simulink model "lab3"  (R2021b)
settings: Solver=VariableStepAuto  StartTime=0.0  StopTime=700  RelTol=1e-3
undefined symbols (not defined in the file): c, J, kb, kt, L, R
libraries: simulink x5, slpidlib x1
settings Model: Creator=Venik  LastModifiedBy=Venik

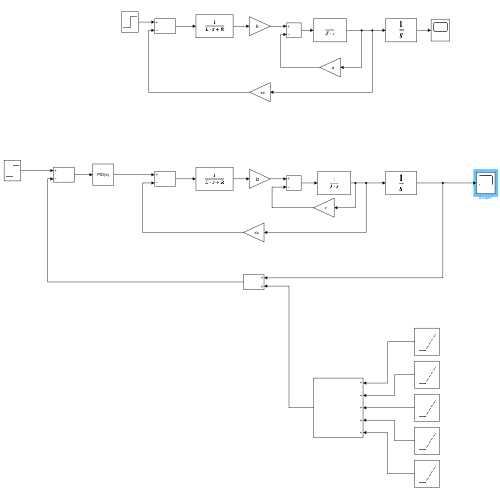
[thumbnail: Simulink's stored preview of the top-level diagram]
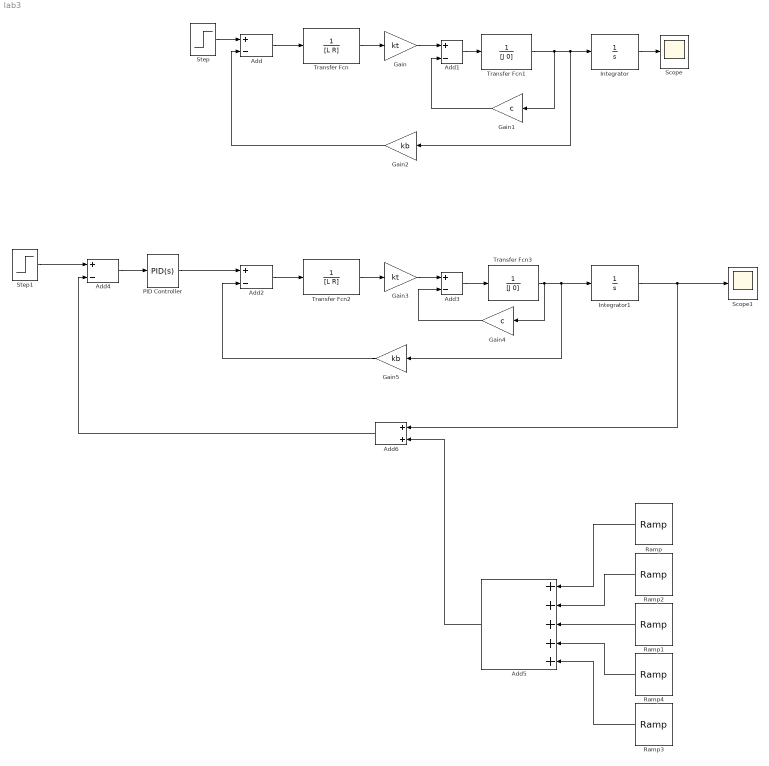
== system lab3 ==
  Add{,1..4} (5 alike) : Sum  Inputs=+-
  Add5 : Sum  Inputs=+++++
  Add6 : Sum
  Gain : Gain  Gain=kt
  Gain1 : Gain  Gain=c
  Gain2 : Gain  Gain=kb
  Gain3 : Gain  Gain=kt
  Gain4 : Gain  Gain=c
  Gain5 : Gain  Gain=kb
  Integrator : Integrator
  Integrator1 : Integrator
  PID Controller : slpidlib/PID Controller  Controller=PID  Form=Parallel  TimeDomain=Continuous-time  UseExternalTs=off  SampleTime=-1  IntegratorMethod=Forward Euler  FilterMethod=Forward Euler  ControllerParametersSource=internal  P=2  I=0.1  D=10  UseFilter=on  N=100  TunerSelectOption=Transfer Function Based (PID Tuner App)  InitialConditionSource=internal  InitialConditionForIntegrator=0  InitialConditionForFilter=0  DifferentiatorICPrevScaledInput=0  ExternalReset=none  TrackingMode=off  Kt=1  LimitOutput=off  SatLimitsSource=internal  UpperSaturationLimit=inf  LowerSaturationLimit=-inf  LinearizeAsGain=on  AntiWindupMode=none  Kb=1  POutMin=[]  POutMax=[]  IOutMin=[]  IOutMax=[]  DOutMin=[]  DOutMax=[]  NOutMin=[]  NOutMax=[]  SumOutMin=[]  SumOutMax=[]  SaturationOutMin=[]  SaturationOutMax=[]  PParamMin=[]  PParamMax=[]  IParamMin=[]  IParamMax=[]  DParamMin=[]  DParamMax=[]  NParamMin=[]  NParamMax=[]  KbParamMin=[]  KbParamMax=[]  KtParamMin=[]  KtParamMax=[]  KbOutMin=[]  KbOutMax=[]  KtOutMin=[]  KtOutMax=[]  IntegratorOutMin=[]  IntegratorOutMax=[]  FilterOutMin=[]  FilterOutMax=[]  SumI1OutMin=[]  SumI1OutMax=[]  SumI2OutMin=[]  SumI2OutMax=[]  SumI3OutMin=[]  SumI3OutMax=[]  SumI4OutMin=[]  SumI4OutMax=[]  SumDOutMin=[]  SumDOutMax=[]  DifferentiatorOutMin=[]  DifferentiatorOutMax=[]  FilterDiffOutCoefMin=[]  FilterDiffOutCoefMax=[]  ReciprocalOutMin=[]  ReciprocalOutMax=[]  SumDenOutMin=[]  SumDenOutMax=[]  SumNumOutMin=[]  SumNumOutMax=[]  DivideOutMin=[]  DivideOutMax=[]  UdiffTsProdOutMin=[]  UdiffTsProdOutMax=[]  NTsProdOutMin=[]  NTsProdOutMax=[]  UintegralTsProdOutMin=[]  UintegralTsProdOutMax=[]  UngainTsProdOutMin=[]  UngainTsProdOutMax=[]  IntegratorContinuousStateAttributes=''  IntegratorStateMustResolveToSignalObject=off  IntegratorRTWStateStorageClass=Auto  FilterContinuousStateAttributes=''  FilterStateMustResolveToSignalObject=off  FilterRTWStateStorageClass=Auto  ParallelPVariant=InternalParameters  IdealPVariant=Disabled  IVariant=InternalParameters  DVariant=InternalParameters  IntegratorVariant=Continuous  SatVariant=Disabled  AWVariant=Passthrough  PCopyVariant=Disabled  TRVariant=Disabled  FdbkBlocksVariant=Forward  IdealPFdbkVariant=Disabled  SatFdbkVariant=Disabled  DerivativeFilterVariant=ContFilter  NVariant=InternalParameters  NCopyVariant=Disabled  FilterICVariant=InternalICsFilter  IntegratorICVariant=InternalICs  ExternalResetVariant=Disabled  TRSumVariant=Passthrough  SumFdbkVariant=Disabled  SumVariant=Sum_PID  TsampFilterVariant=InternalTs  TsampNgainVariant=Passthrough  TsampIntegralVariant=Passthrough  ExternalSaturationOutDataTypeStr=Inherit: Same as second input
  Ramp : simulink/Sources/Ramp  slope=0  start=0  InitialOutput=0
  Ramp1 : simulink/Sources/Ramp  slope=-0.2  start=170  InitialOutput=0
  Ramp2 : simulink/Sources/Ramp  slope=0.2  start=150  InitialOutput=0
  Ramp3 : simulink/Sources/Ramp  slope=0.1  start=350  InitialOutput=0
  Ramp4 : simulink/Sources/Ramp  slope=-0.1  start=300  InitialOutput=0
  Scope : Scope
  Scope1 : Scope
  Step : Step  After=3  SampleTime=0
  Step1 : Step  After=3  SampleTime=0
  Transfer Fcn : TransferFcn  Denominator=[L R]
  Transfer Fcn1 : TransferFcn  Denominator=[J 0]
  Transfer Fcn2 : TransferFcn  Denominator=[L R]
  Transfer Fcn3 : TransferFcn  Denominator=[J 0]
  wires:
  Add/1 -> Transfer Fcn/1
  Transfer Fcn/1 -> Gain/1
  Gain/1 -> Add1/1
  Transfer Fcn1/1 -> Gain1/1, Gain2/1, Integrator/1
  Add1/1 -> Transfer Fcn1/1
  Gain1/1 -> Add1/2
  Gain2/1 -> Add/2
  Integrator/1 -> Scope/1
  Step/1 -> Add/1
  PID Controller/1 -> Add2/1
  Add2/1 -> Transfer Fcn2/1
  Transfer Fcn2/1 -> Gain3/1
  Gain4/1 -> Add3/2
  Integrator1/1 -> Add6/1, Scope1/1
  Gain5/1 -> Add2/2
  Gain3/1 -> Add3/1
  Add3/1 -> Transfer Fcn3/1
  Transfer Fcn3/1 -> Integrator1/1, Gain5/1, Gain4/1
  Add4/1 -> PID Controller/1
  Add6/1 -> Add4/2
  Step1/1 -> Add4/1
  Ramp/1 -> Add5/1
  Ramp2/1 -> Add5/2
  Ramp1/1 -> Add5/3
  Ramp4/1 -> Add5/4
  Ramp3/1 -> Add5/5
  Add5/1 -> Add6/2
